simulink model "part1"  (R2023b)
settings: Solver=VariableStepAuto  StartTime=0.0  StopTime=100  RelTol=1e-3
undefined symbols (not defined in the file): gray
libraries: visiongeotforms x2, visiontextngfix x1, visionsources x1
settings Model: Creator=10373  LastModifiedBy=10373

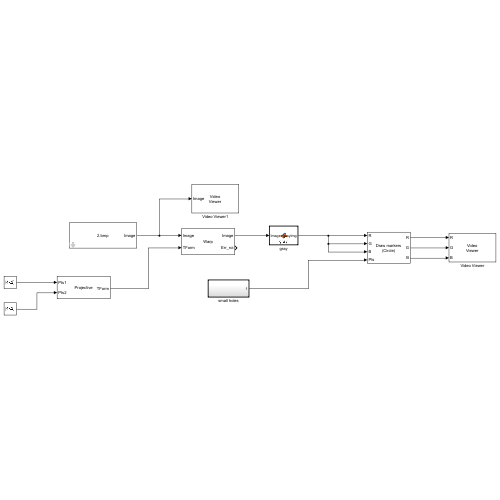
[thumbnail: Simulink's stored preview of the top-level diagram]
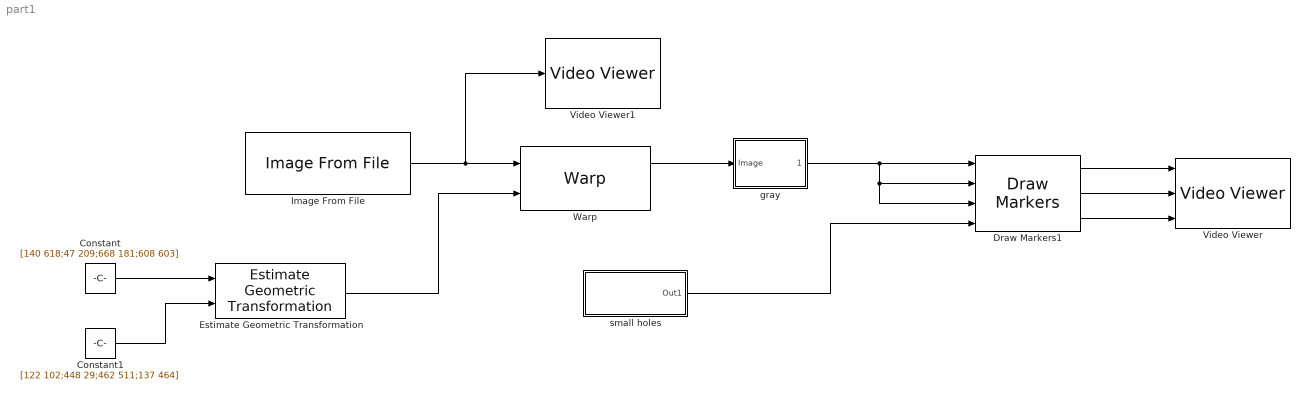
== system part1 ==
  Constant : Constant  Value=[140 618;47 209;668 181;608 603]
  Constant1 : Constant  Value=[122 102;448 29;462 511;137 464]
  Draw Markers1 : visiontextngfix/Draw Markers  shape=Circle  size=3  fill=off  fillClrSource=Specify via dialog  display=User-specified value  intensity=200  color=[255 0 0]  opacity=0.6  viewport=Entire image  antialiasing=off  inType=Obsolete  imagePorts=Separate color signals  roundingMode=Floor  overflowMode=off  memoryMode=Specify word length  memoryWordLength=16  memoryFracLength=15  prodOutputMode=Binary point scaling  prodOutputWordLength=32  prodOutputFracLength=14
  Estimate Geometric Transformation : visiongeotforms/Estimate Geometric Transformation  tformType=Projective  isRandomSampling=on  algMethod=Random Sample Consensus (RANSAC)  distanceAlg=2.5  distanceGeo=2.5  numMethod=Specified value  sampleNum=500  desiredConfidence=99  maxSampleNum=1000  isStopSampling=off  percentStop=75  isRefineTForm=off  isReleaseMode=on  isOutputInlier=off  outDT4IntInput=Obsolete10a  outDT4IntInputActive=Single  isVarSizeAllowed=on
  Image From File : visionsources/Image From File  Tag=vipblks_nd  FileName=D:\Homework\Digital Image\lab2\PCB\2.bmp  Ts=inf  imagePorts=One multidimensional signal  OutPortLabels=R|G|B  ImageDataType=double  sdImageDataType=uint(8)  Signed=on  WordLength=16  FractionLengthMode=User-defined  FractionLength=15
  Video Viewer : VideoViewer  imagePorts=separate color signals  colormapValue=gray(256)  FigPos=[-129.666666666667 954.666666666667 1706.66666666667 814.666666666667]
  Video Viewer1 : VideoViewer  colormapValue=gray(256)  FigPos=[249.666666666667 793.333333333333 908.666666666667 628.666666666667]
  Warp : visiongeotforms/Warp  TransformMatrixSource=Input port  TransformMatrix=eye( 3 )  InterpolationMethod=Bilinear  BackgroundFillValue=0  OutputImagePositionSource=Same as input image  OutputImagePosition=[ 1, 1, 512, 512 ]  ROIInputPort=off  ROIValidityOutputPort=on  SimulateUsing=Interpreted execution
  gray : MATLAB Function  TreatAsAtomicUnit=on
  small holes : Subsystem  TreatAsAtomicUnit=on
  wires:
  Constant/1 -> Estimate Geometric Transformation/1
  Constant1/1 -> Estimate Geometric Transformation/2
  Image From File/1 -> Video Viewer1/1, Warp/1
  Estimate Geometric Transformation/1 -> Warp/2
  Draw Markers1/1 -> Video Viewer/1
  Warp/1 -> gray/1(Image)
  Draw Markers1/2 -> Video Viewer/2
  Draw Markers1/3 -> Video Viewer/3
  gray/1(grayImg) -> Draw Markers1/3, Draw Markers1/2, Draw Markers1/1
  small holes/1(Out1) -> Draw Markers1/4

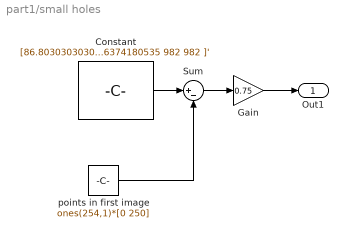
== system part1/small holes ==
  Constant : Constant  Value=|
      | [86.8030303030303	86.8030303030303	227.219696969697	227.219696969697	271.897727272727	297.428030303030	374.018939393939	374.018939393939	374.018939393939	374.018939393939	374.018939393939	374.018939393939	412.314393939394	488.905303030303	527.200757575758	527.200757575758	527.200757575758	527.200757575758	527.200757575758	527.200757575758	533.583333333333	508.053030303030	482.522727272727	456.992424242424	431.462121212121	393.166666666667	393.166666666667	393.166666666667	393.166666666667	431.462121212121	456.992424242424	482.522727272727	508.053030303030	533.583333333333	559.113636363636	584.643939393939	610.174242424242	597.409090909091	571.878787878788	533.583333333333	508.053030303030	469.757575757576	444.227272727273	559.113636363636	584.643939393939	610.174242424242	342.106060606061	342.106060606061	616.556818181818	514.435606060606	527.200757575758	527.200757575758	527.200757575758	527.200757575758	527.200757575758	527.200757575758	527.200757575758	527.200757575758	527.200757575758	527.200757575758	527.200757575758	527.200757575758	527.200757575758	527.200757575758	488.905303030303	488.905303030303	488.905303030303	488.905303030303	488.905303030303	488.905303030303	458.905303030303	488.905303030303	488.905303030303	488.905303030303	488.905303030303	488.905303030303	488.905303030303	412.314393939394	412.314393939394	412.314393939394	412.314393939394	412.314393939394	412.314393939394	412.314393939394	412.314393939394	412.314393939394	412.314393939394	412.314393939394	412.314393939394	412.314393939394	374.018939393939	374.018939393939	374.018939393939	374.018939393939	374.018939393939	374.018939393939	374.018939393939	374.018939393939	374.018939393939	374.018939393939	374.018939393939	374.018939393939	374.018939393939	374.018939393939	342.106060606061	342.106060606061	342.106060606061	342.106060606061	342.106060606061	610.174242424242	610.174242424242	291.045454545455	291.045454545455	271.897727272727	259.132575757576	233.602272727273	214.454545454545	214.454545454545	214.454545454545	233.602272727273	214.454545454545	214.454545454545	233.602272727273	214.454545454545	214.454545454545	233.602272727273	259.132575757576	291.045454545455	316.575757575758	291.045454545455	271.897727272727	291.045454545455	291.045454545455	291.045454545455	316.575757575758	316.575757575758	316.575757575758	271.897727272727	271.897727272727	220.837121212121	220.837121212121	220.837121212121	246.367424242424	271.897727272727	297.428030303030	316.575757575758	157.011363636364	131.481060606061	99.5681818181818	74.0378787878788	144.246212121212	169.776515151515	182.541666666667	182.541666666667	437.844696969697	539.965909090909	150.628787878788	150.628787878788	254.026515151515	233.602272727273	213.178030303030	223.390151515152	243.814393939394	264.238636363636	148.841666666667	176.669696969697	204.497727272727	232.325757575758	218.539393939394	190.711363636364	162.883333333333	135.055303030303	118.715909090909	256.367424242424	246.367424242424	291.045454545455	316.575757575758	316.575757575758	291.045454545455	342.106060606061	342.106060606061	559.113636363636	584.643939393939	610.174242424242	610.174242424242	584.643939393939	559.113636363636	648.469696969697	648.469696969697	648.469696969697	648.469696969697	648.469696969697	648.469696969697	648.469696969697	674	674	674	674	674	674	674	674	674	674	674	648.469696969697	648.469696969697	648.469696969697	674	674	648.469696969697	648.469696969697	648.469696969697	648.469696969697	674	674	648.469696969697	648.469696969697	648.469696969697	648.469696969697	648.469696969697	648.469696969697	674	674	674	674	674	610.174242424242	584.643939393939	559.113636363636	565.496212121212	591.026515151515	584.643939393939	610.174242424242	559.113636363636	565.496212121212	591.026515151515	591.026515151515	565.496212121212	488.905303030303	463.375000000000	437.844696969697	342.106060606061	316.575757575758	291.045454545455	125.098484848485	99.5681818181818	74.0378787878788	591.026515151515	565.496212121212	400.315151515152	334.957575757576	334.957575757576	400.315151515152
      | ;497.685325264750	547.206253151790	522.445789208270	472.924861321230	429.594049420071	429.594049420071	423.403933434191	448.164397377711	472.924861321230	497.685325264750	522.445789208270	547.206253151790	534.826021180030	534.826021180030	547.206253151790	522.445789208270	497.685325264750	472.924861321230	448.164397377711	423.403933434191	392.453353504791	392.453353504791	392.453353504791	392.453353504791	392.453353504791	392.453353504791	367.692889561271	330.552193645991	305.791729702471	318.171961674231	318.171961674231	318.171961674231	318.171961674231	318.171961674231	318.171961674231	318.171961674231	318.171961674231	287.221381744831	287.221381744831	287.221381744831	287.221381744831	287.221381744831	287.221381744831	392.453353504791	392.453353504791	392.453353504791	485.305093292990	510.065557236510	930.993444276349	930.993444276349	893.852748361069	869.092284417549	844.331820474029	819.571356530509	794.810892586989	770.050428643469	745.289964699950	720.529500756430	695.769036812910	671.008572869390	646.248108925870	621.487644982350	596.727181038830	571.966717095310	559.586485123550	584.346949067070	609.107413010590	633.867876954110	658.628340897630	683.388804841150	708.149268784670	732.909732728190	757.670196671710	782.430660615230	807.191124558749	831.951588502269	856.712052445789	856.712052445789	831.951588502269	807.191124558749	782.430660615230	757.670196671710	732.909732728190	708.149268784670	683.388804841150	658.628340897630	633.867876954110	609.107413010590	584.346949067070	559.586485123550	571.966717095310	596.727181038830	621.487644982350	646.248108925870	671.008572869390	695.769036812910	720.529500756430	745.289964699950	770.050428643469	794.810892586989	819.571356530509	844.331820474029	869.092284417549	893.852748361069	893.852748361069	794.810892586989	770.050428643469	671.008572869390	565.776601109430	671.008572869390	695.769036812910	695.769036812910	720.529500756430	720.529500756430	695.769036812910	695.769036812910	695.769036812910	720.529500756430	745.289964699950	745.289964699950	770.050428643469	794.810892586989	794.810892586989	819.571356530509	844.331820474029	844.331820474029	844.331820474029	844.331820474029	844.331820474029	819.571356530509	819.571356530509	794.810892586989	770.050428643469	745.289964699950	745.289964699950	658.628340897630	633.867876954110	633.867876954110	658.628340897630	658.628340897630	609.107413010590	565.776601109430	565.776601109430	565.776601109430	565.776601109430	565.776601109430	677.198688855270	677.198688855270	677.198688855270	677.198688855270	726.719616742310	726.719616742310	770.050428643469	869.092284417549	961.944024205749	961.944024205749	472.924861321230	522.445789208270	900.042864346949	900.042864346949	900.042864346949	924.803328290469	924.803328290469	924.803328290469	361.502773575391	361.502773575391	361.502773575391	361.502773575391	386.263237518911	386.263237518911	386.263237518911	386.263237518911	435.784165405951	415.784165405951	386.263237518911	460.544629349471	460.544629349471	534.826021180030	534.826021180030	534.826021180030	460.544629349471	510.065557236510	510.065557236510	510.065557236510	547.206253151790	547.206253151790	547.206253151790	547.206253151790	522.445789208270	497.685325264750	472.924861321230	448.164397377711	423.403933434191	398.643469490671	398.643469490671	423.403933434191	448.164397377711	472.924861321230	497.685325264750	522.445789208270	547.206253151790	695.769036812910	671.008572869390	646.248108925870	621.487644982350	621.487644982350	596.727181038830	571.966717095310	571.966717095310	596.727181038830	646.248108925870	671.008572869390	695.769036812910	720.529500756430	720.529500756430	745.289964699950	745.289964699950	770.050428643469	794.810892586989	819.571356530509	844.331820474029	869.092284417549	899.092284417549	844.331820474029	819.571356530509	794.810892586989	770.050428643469	745.289964699950	745.289964699950	745.289964699950	794.810892586989	794.810892586989	831.951588502269	831.951588502269	831.951588502269	869.092284417549	869.092284417549	906.232980332829	906.232980332829	924.803328290469	924.803328290469	924.803328290469	596.727181038830	596.727181038830	596.727181038830	708.149268784670	708.149268784670	708.149268784670	955.753908219869	955.753908219869	937.926374180535	937.926374180535	982	982
      | ]'
  Gain : Gain  Gain=0.75
  Sum : Sum  Inputs=|+-
  points in first image : Constant  Value=ones(254,1)*[0 250]  VectorParams1D=off  OutDataTypeStr=single
  Out1 : Outport
  wires:
  Gain/1 -> Out1/1
  points in first image/1 -> Sum/2
  Sum/1 -> Gain/1
  Constant/1 -> Sum/1

== matlab function part1/gray ==
  data: Image input; grayImg output
function grayImg = gray(Image)

grayImg = rgb2gray(Image);%灰度化
% SImg = imadjust(grayImg);%饱和度处理


end
